simulink model "VCU10"  (R2021b)
settings: Solver=FixedStepDiscrete  StartTime=0.0  StopTime=10.0  FixedStep=0.01  RelTol=1e-3
values from neighbouring files (symbols this model uses):
  F = 0.0    [VCU10DB.sldd]
  FSEC_ESP_EMERGENCY_PRESSURE_MPA = 8.0    [VCU10DB.sldd]
  T = 1.0    [VCU10DB.sldd]
libraries: simulink x148, hdlsllib x90
(part 2 of 4)

== system VCU10/Motor_Control ==
  note: AS torque enable = ASMS AND AS_Driving AND R2D complete AND no Emergency lock.
  sensor_signal : Inport
  manual_driving_flag : Inport  Port=2
  as_flag : Inport  Port=3
  ipc_motor_torque : Inport  Port=4
  ts : Inport  Port=5
  function : TriggerPort  TriggerType=function-call  VariantControl=(inherit)
  ASTorque_Calculation : Subsystem
  AS_Driving_Read : DataStoreRead  DataStoreName=as_driving_flag  IndexOptions=Index vector (dialog)  Indices=1  OutputSizes=1
  AS_Emergency_Read : DataStoreRead  DataStoreName=as_emergency_flag  IndexOptions=Index vector (dialog)  Indices=1  OutputSizes=1
  AS_Torque_Enable : Logic  Inputs=4  AllPortsSameDT=off  OutDataTypeStr=boolean
  Emergency_Torque_Gate : Switch  Threshold=0.5
  Emergency_Zero_Torque : Constant  Value=0  OutDataTypeStr=double
  FSEC_Safety_Lock_Read : DataStoreRead  DataStoreName=safety_lock  IndexOptions=Index vector (dialog)  Indices=1  OutputSizes=1
  MCU1_Rx_Command : Subsystem
  MCU1_Rx_Command3 : Subsystem
  ManualTorque_Calculation : Subsystem
  Motor_Torque_Stateflow : Stateflow chart  TreatAsAtomicUnit=on
      settings: PortSchema="{\"entries\":[{\"content\":{\"sides\":[{\"content\":{\"connectorIds\":[\"In1\",\"In3\",\"In2\",\"In4\"]},\"type\":\"ConnectorPlacement.EquallySpacedRectSide\",\"uuid\":\"d9a8263c-4b6f-42da-8ac2-d6351ac22d7e\"},{\"content\":{\"connectorIds\":[\"Out1\"],\"side\":\"RIGHT\"},\"type\":\"ConnectorPlacement.EquallySpacedRectSide\",\"uuid\":\"5afddd84-d4d9-4932-bab9-0cf7e7557aa2\"},{\"content\":{\"connectorIds\":[],\"side\":\"TOP\"},\"type\":\"ConnectorPlacement.EquallySpacedRectSide\",\"uuid\":\"31244ac9-97b6-45b3-a8be-c5389c850836\"}]},\"type\":\"ConnectorPlacement.EquallySpacedConnector\",\"uuid\":\"4a9ac252-b735-4ae7-9487-f10bc9e5bec6\"}],\"packageUris\":[\"http://schema.mathworks.com/mf0/Connector/R2020b\"],\"version\":\"1.0\"}"
  No_FSEC_Safety_Lock : Logic  Operator=NOT  Inputs=1  AllPortsSameDT=off  OutDataTypeStr=boolean
  R2D_Complete : Logic  Operator=NOT  Inputs=1  AllPortsSameDT=off  OutDataTypeStr=boolean
  R2D_Read : DataStoreRead  DataStoreName=r2d_flag  IndexOptions=Index vector (dialog)  Indices=1  OutputSizes=1
  cana_motor_cmd : Outport
  cana_motor_cmd3 : Outport  Port=2
  wires:
  sensor_signal/1 -> ManualTorque_Calculation/1(sensor_signal)
  manual_driving_flag/1 -> Motor_Torque_Stateflow/1(manual_driving_flag)
  ManualTorque_Calculation/1(manual_torque) -> Motor_Torque_Stateflow/3(manual_torque)
  ASTorque_Calculation/1(as_torque) -> Motor_Torque_Stateflow/4(as_torque)
  ts/1 -> MCU1_Rx_Command/1(ts)
  [motor_torque] -> MCU1_Rx_Command/2(motor_torque)
  MCU1_Rx_Command/1(cana_motor_cmd) -> cana_motor_cmd/1
  MCU1_Rx_Command3/1(cana_motor_cmd3) -> cana_motor_cmd3/1
  ipc_motor_torque/1 -> ASTorque_Calculation/1(ipc_motor_torque)
  Emergency_Zero_Torque/1 -> Emergency_Torque_Gate/1
  AS_Emergency_Read/1 -> Emergency_Torque_Gate/2
  Motor_Torque_Stateflow/1(motor_torque) -> Emergency_Torque_Gate/3
  Emergency_Torque_Gate/1 -> [motor_torque]
  R2D_Read/1 -> R2D_Complete/1
  FSEC_Safety_Lock_Read/1 -> No_FSEC_Safety_Lock/1
  as_flag/1 -> AS_Torque_Enable/1
  AS_Driving_Read/1 -> AS_Torque_Enable/2
  R2D_Complete/1 -> AS_Torque_Enable/3
  No_FSEC_Safety_Lock/1 -> AS_Torque_Enable/4
  AS_Torque_Enable/1 -> Motor_Torque_Stateflow/2(as_task)

== system VCU10/Output_Convert ==
  note: Hardware mapping (netlist 2026-07-30): OUT1..7 = Brake, ASSI-B, ASSI-Y, EBS error, RES error, reserved, reserved; HO1..8 = EBS trigger, BMS, IMD, DI8, RUN, R2D, Emergency, reserved.
  led_brake : Inport
  led_assi_y : Inport  Port=2
  led_assi_b : Inport  Port=3
  led_ebserror : Inport  Port=4
  res_error : Inport  Port=5
  ebs_trig : Inport  Port=6
  led_bmserr : Inport  Port=7
  led_imderr : Inport  Port=8
  di8 : Inport  Port=9
  run : Inport  Port=10
  buzzer_r2d : Inport  Port=11
  buzzer_ebs : Inport  Port=12
  function : TriggerPort  TriggerType=function-call  VariantControl=(inherit)
  Physical_HO1_8_Pack : hdlsllib/Logic and Bit Operations/Bit Concat  numInputs=8
  Physical_OUT1_7_Pack : hdlsllib/Logic and Bit Operations/Bit Concat  numInputs=7
  Unused_HO_Bit : Constant  Value=false  OutDataTypeStr=boolean
  Unused_OUT_Bit : Constant  Value=false  OutDataTypeStr=boolean
  model_lox : Outport
  model_hox : Outport  Port=2
  wires:
  Unused_OUT_Bit/1 -> Physical_OUT1_7_Pack/1, Physical_OUT1_7_Pack/2
  res_error/1 -> Physical_OUT1_7_Pack/3
  led_ebserror/1 -> Physical_OUT1_7_Pack/4
  led_assi_y/1 -> Physical_OUT1_7_Pack/5
  led_assi_b/1 -> Physical_OUT1_7_Pack/6
  led_brake/1 -> Physical_OUT1_7_Pack/7
  Physical_OUT1_7_Pack/1 -> model_lox/1  "model_lox"
  Unused_HO_Bit/1 -> Physical_HO1_8_Pack/1
  buzzer_ebs/1 -> Physical_HO1_8_Pack/2
  buzzer_r2d/1 -> Physical_HO1_8_Pack/3
  run/1 -> Physical_HO1_8_Pack/4
  di8/1 -> Physical_HO1_8_Pack/5
  led_imderr/1 -> Physical_HO1_8_Pack/6
  led_bmserr/1 -> Physical_HO1_8_Pack/7
  ebs_trig/1 -> Physical_HO1_8_Pack/8
  Physical_HO1_8_Pack/1 -> model_hox/1  "model_hox"

== system VCU10/Res ==
  res_msg : Inport
  function : TriggerPort  TriggerType=function-call  VariantControl=(inherit)
  Bus Selector : BusSelector  OutputSignals=res_stop
  Res_Msg : Subsystem
  res_signal : Outport
  res_error : Outport  Port=2
  wires:
  res_msg/1 -> Res_Msg/1(res_msg)
  Res_Msg/1(res_signal) -> Bus Selector/1, res_signal/1
  Bus Selector/1 -> res_error/1  "<res_stop>"

== system VCU10/Sensor_Signal ==
  note: EBS气缸侧气压
  note: EBS气瓶侧气压
  note: FSEC diagnostics: brkps_raw is checked against 0.10-4.90 V. Air pressure sensor 1 is the reservoir/ready side; sensor 2 is the solenoid downstream/cylinder side.
  apps1 : Inport
  apps2 : Inport  Port=2
  brkps : Inport  Port=3
  airprs_sensor1 : Inport  Port=4
  airprs_sensor2 : Inport  Port=5
  wlspd_fsensor : Inport  Port=6
  wlspd_hsensor : Inport  Port=7
  function : TriggerPort  TriggerType=function-call  VariantControl=(inherit)
  1-D Lookup Table : Lookup_n-D  NumberOfTableDimensions=1  BreakpointsForDimension1=[252 2000]  IndexSearchMethod=Linear search  Table=[0.0 1.0]  ExtrapMethod=Clip  UseLastTableValue=on  InternalRulePriority=Speed  OutDataTypeStr=double  RndMeth=Simplest  InputSameDT=on
  1-D Lookup Table1 : Lookup_n-D  NumberOfTableDimensions=1  BreakpointsForDimension1=[252 2000]  IndexSearchMethod=Linear search  Table=[0.0 1.0]  ExtrapMethod=Clip  UseLastTableValue=on  InternalRulePriority=Speed  OutDataTypeStr=double  RndMeth=Simplest  InputSameDT=on
  1-D Lookup Table9 : Lookup_n-D  NumberOfTableDimensions=1  BreakpointsForDimension1=[252 2000]  IndexSearchMethod=Linear search  Table=[0.0 1.0]  ExtrapMethod=Clip  UseLastTableValue=on  InternalRulePriority=Speed  OutDataTypeStr=double  RndMeth=Simplest  InputSameDT=on
  Bus Creator : BusCreator  Inputs=12
  Data Type Conversion{,1..9,12,15} (12 alike) : DataTypeConversion  OutDataTypeStr=double
  Gain : Gain  Gain=single(0.001)
  Gain1 : Gain  Gain=single(0.001)
  Saturation : Saturate  UpperLimit=1  LowerLimit=0
  Saturation1 : Saturate  UpperLimit=1  LowerLimit=0
  Saturation2 : Saturate  UpperLimit=1  LowerLimit=0
  Subsystem : Subsystem
  sensor_signal : Outport
  wires:
  apps1/1 -> Data Type Conversion1/1, 1-D Lookup Table/1
  1-D Lookup Table/1 -> Data Type Conversion/1
  Data Type Conversion/1 -> Saturation/1
  Saturation/1 -> Bus Creator/1  "apps1_01"
  Data Type Conversion1/1 -> Bus Creator/2  "apps1_raw"
  Data Type Conversion2/1 -> Saturation1/1
  apps2/1 -> 1-D Lookup Table9/1, Data Type Conversion3/1
  1-D Lookup Table9/1 -> Data Type Conversion2/1
  Saturation1/1 -> Bus Creator/3  "apps2_01"
  Data Type Conversion3/1 -> Bus Creator/4  "apps2_raw"
  brkps/1 -> 1-D Lookup Table1/1, Data Type Conversion5/1
  1-D Lookup Table1/1 -> Data Type Conversion4/1
  Data Type Conversion4/1 -> Saturation2/1
  Saturation2/1 -> Bus Creator/5  "brkps"
  Data Type Conversion5/1 -> Bus Creator/6  "brkps_raw"
  wlspd_fsensor/1 -> Data Type Conversion6/1
  Data Type Conversion6/1 -> Subsystem/1(f_frequency)
  wlspd_hsensor/1 -> Data Type Conversion7/1
  Data Type Conversion7/1 -> Subsystem/2(h_frequency)
  Subsystem/1(wheel_speed_f) -> Data Type Conversion8/1
  Subsystem/2(wheel_speed_h) -> Data Type Conversion9/1
  Data Type Conversion8/1 -> Bus Creator/7  "wlspd_fsensor"
  Data Type Conversion9/1 -> Bus Creator/8  "wlspd_hsensor"
  Bus Creator/1 -> sensor_signal/1
  Data Type Conversion12/1 -> Bus Creator/9  "airprs_sensor1"
  airprs_sensor2/1 -> Gain1/1, Bus Creator/12  "airprs2_raw"
  Data Type Conversion15/1 -> Bus Creator/10  "airprs_sensor2"
  airprs_sensor1/1 -> Gain/1, Bus Creator/11  "airprs1_raw"
  Gain/1 -> Data Type Conversion12/1
  Gain1/1 -> Data Type Conversion15/1

== system VCU10/TS_Activation ==
  note: Software Emergency lock forces TS=0 until VCU low-voltage power cycle.
  note: AS Emergency forces TS=0 in the same model step; the software lock keeps TS off until VCU low-voltage power cycle.
  di8_out : Inport
  run_button : Inport  Port=2
  tsms_button : Inport  Port=3
  di8_in : Inport  Port=4
  as_flag : Inport  Port=5
  brake_on : Inport  Port=6
  function : TriggerPort  TriggerType=function-call  VariantControl=(inherit)
  AS_Emergency_Read : DataStoreRead  DataStoreName=as_emergency_flag  IndexOptions=Index vector (dialog)  Indices=1  OutputSizes=1
  Chart : Stateflow chart  TreatAsAtomicUnit=on
  Chart1 : Stateflow chart  TreatAsAtomicUnit=on
  Chart2 : Stateflow chart  TreatAsAtomicUnit=on
  FSEC_Safety_Lock_Read : DataStoreRead  DataStoreName=safety_lock  IndexOptions=Index vector (dialog)  Indices=1  OutputSizes=1
  Logical Operator : Logic  Operator=NOT  AllPortsSameDT=off  OutDataTypeStr=boolean
  Logical Operator1 : Logic  Operator=NOT  AllPortsSameDT=off  OutDataTypeStr=boolean
  Logical Operator2 : Logic  Operator=NOT  AllPortsSameDT=off  OutDataTypeStr=boolean
  No_AS_Emergency : Logic  Operator=NOT  Inputs=1  AllPortsSameDT=off  OutDataTypeStr=boolean
  No_FSEC_Safety_Lock : Logic  Operator=NOT  Inputs=1  AllPortsSameDT=off  OutDataTypeStr=boolean
  Switch : Switch  Criteria=u2 > Threshold
  TS_Safety_Gate : Logic  Inputs=3  AllPortsSameDT=off  OutDataTypeStr=boolean
  ts : Outport
  di8 : Outport  Port=2
  run : Outport  Port=3
  ts_warning : Outport  Port=4  OutDataTypeStr=boolean
  wires:
  di8_out/1 -> Logical Operator/1
  run_button/1 -> Logical Operator1/1
  Logical Operator1/1 -> Chart1/1(run_button)
  Chart/1(di8) -> di8/1, Chart2/1(di8)  "di8"
  Chart1/1(run) -> run/1, Chart2/2(run)  "run"
  tsms_button/1 -> Chart2/3(tsms_button)
  brake_on/1 -> Chart2/4(brake_on)
  as_flag/1 -> Chart2/5(as_flag), Switch/2
  di8_in/1 -> Logical Operator2/1
  Logical Operator/1 -> Switch/1
  Logical Operator2/1 -> Switch/3
  Switch/1 -> Chart/1(di8_button)
  Chart2/2(ts_warning) -> ts_warning/1
  FSEC_Safety_Lock_Read/1 -> No_FSEC_Safety_Lock/1
  Chart2/1(ts) -> TS_Safety_Gate/1
  No_FSEC_Safety_Lock/1 -> TS_Safety_Gate/2
  AS_Emergency_Read/1 -> No_AS_Emergency/1
  No_AS_Emergency/1 -> TS_Safety_Gate/3
  TS_Safety_Gate/1 -> ts/1

== system VCU10/AMI_CAN/AMI_Receivemsg ==
  AMI_Tx : Inport
  Bit Shift : hdlsllib/Logic and Bit Operations/Bit Shift  mode=Shift Right Logical  N=4
  Bitwise AND : simulink/Logic and Bit Operations/Bitwise Operator  logicop=AND  UseBitMask=on  BitMask=bin2dec('11110000')  BitMaskRealWorld=Stored Integer
  Demux : Demux  Outputs=8
  Terminator{,1..6} (7 alike) : Terminator
  ami_astask : Outport
  wires:
  Demux/6 -> Terminator3/1
  Demux/2 -> Terminator6/1
  Demux/4 -> Terminator1/1
  AMI_Tx/1 -> Demux/1
  Demux/7 -> Terminator4/1
  Demux/5 -> Terminator2/1
  Demux/8 -> Terminator5/1
  Demux/3 -> Terminator/1
  Demux/1 -> Bitwise AND/1
  Bitwise AND/1 -> Bit Shift/1
  Bit Shift/1 -> ami_astask/1

== system VCU10/AMI_CAN/AMI_Transmitmsg ==
  as_flag_state : Inport
  task_finish : Inport  Port=2
  Add1 : Sum
  Bit Shift : hdlsllib/Logic and Bit Operations/Bit Shift  mode=Shift Left Logical  N=1
  Bitwise AND : simulink/Logic and Bit Operations/Bitwise Operator  logicop=AND  UseBitMask=on  BitMask=bin2dec('01111111')  BitMaskRealWorld=Stored Integer
  Bus Selector : BusSelector  OutputSignals=as_off_flag,manual_driving_flag,as_ready_flag,r2d_flag,as_driving_flag,as_finished_flag,as_emergency_flag
  Chart : Stateflow chart  TreatAsAtomicUnit=on
  Ground{,1..6} (7 alike) : Ground
  Mux : Mux  Inputs=8
  Signal Conversion : SignalConversion  OverrideOpt=off
  AMI_RX : Outport
  wires:
  as_flag_state/1 -> Bus Selector/1
  Bitwise AND/1 -> Bit Shift/1
  Bit Shift/1 -> Add1/1
  task_finish/1 -> Add1/2
  Add1/1 -> Mux/1
  Bus Selector/1 -> Chart/1(as_off_flag)  "<as_off_flag>"
  Bus Selector/2 -> Chart/2(munual_driving_flag)  "<manual_driving_flag>"
  Bus Selector/3 -> Chart/3(as_ready_flag)  "<as_ready_flag>"
  Bus Selector/4 -> Chart/4(r2d_flag)  "<r2d_flag>"
  Bus Selector/5 -> Chart/5(as_driving_flag)  "<as_driving_flag>"
  Bus Selector/6 -> Chart/6(as_finished_flag)  "<as_finished_flag>"
  Bus Selector/7 -> Chart/7(as_emergency_flag)  "<as_emergency_flag>"
  Chart/1(ami_process) -> Bitwise AND/1
  Ground/1 -> Mux/2
  Ground1/1 -> Mux/3
  Ground2/1 -> Mux/4
  Ground3/1 -> Mux/5
  Ground4/1 -> Mux/6
  Ground5/1 -> Mux/7
  Ground6/1 -> Mux/8
  Mux/1 -> Signal Conversion/1
  Signal Conversion/1 -> AMI_RX/1

== system VCU10/ASB_Selfcheck/Brake_Sensor_Check ==
  note: 下四路为有效制动阈值油压
  note: 上四路油压信号阈值为非制动状态油压
  note: 所有常数待定
  airprs_sensor1 : Inport
  oilprs_frsensor : Inport  Port=2
  oilprs_rrsensor : Inport  Port=3
  oilprs_flsensor : Inport  Port=4
  oilprs_rlsensor : Inport  Port=5
  Compare To Constant : simulink/Logic and Bit Operations/Compare To Constant  relop=>=  const=3.5  OutDataTypeStr=boolean
  Compare To Constant{1,3,5,7} (4 alike) : simulink/Logic and Bit Operations/Compare To Constant  relop=>=  const=0.848  OutDataTypeStr=boolean
  Compare To Constant{2,4,6,8} (4 alike) : simulink/Logic and Bit Operations/Compare To Constant  relop=>=  const=0.742  OutDataTypeStr=boolean
  Logical Operator : Logic  Inputs=5  AllPortsSameDT=off  OutDataTypeStr=boolean
  Logical Operator1 : Logic  Inputs=4  AllPortsSameDT=off  OutDataTypeStr=boolean
  brksensor_check : Outport
  brake_on : Outport  Port=2
  wires:
  airprs_sensor1/1 -> Compare To Constant/1
  oilprs_frsensor/1 -> Compare To Constant5/1, Compare To Constant1/1
  oilprs_rrsensor/1 -> Compare To Constant7/1, Compare To Constant3/1
  oilprs_flsensor/1 -> Compare To Constant6/1, Compare To Constant2/1
  oilprs_rlsensor/1 -> Compare To Constant8/1, Compare To Constant4/1
  Compare To Constant3/1 -> Logical Operator/3
  Compare To Constant/1 -> Logical Operator/1
  Compare To Constant1/1 -> Logical Operator/2
  Compare To Constant2/1 -> Logical Operator/4
  Compare To Constant4/1 -> Logical Operator/5
  Logical Operator/1 -> brksensor_check/1
  Logical Operator1/1 -> brake_on/1
  Compare To Constant5/1 -> Logical Operator1/1
  Compare To Constant7/1 -> Logical Operator1/2
  Compare To Constant6/1 -> Logical Operator1/3
  Compare To Constant8/1 -> Logical Operator1/4

== system VCU10/AS_Stateflow/Car_Spdzero_Check ==
  wlspd_fsensor : Inport
  wlspd_hsensor : Inport  Port=2
  Compare To Constant : simulink/Logic and Bit Operations/Compare To Constant  relop===  const=0  OutDataTypeStr=boolean
  Compare To Constant1 : simulink/Logic and Bit Operations/Compare To Constant  relop===  const=0  OutDataTypeStr=boolean
  Dead Zone : DeadZone  SaturateOnIntegerOverflow=on
  Dead Zone1 : DeadZone  SaturateOnIntegerOverflow=on
  Logical Operator : Logic  AllPortsSameDT=off  OutDataTypeStr=boolean
  car_spdzero : Outport
  wires:
  wlspd_fsensor/1 -> Dead Zone/1
  wlspd_hsensor/1 -> Dead Zone1/1
  Dead Zone/1 -> Compare To Constant/1
  Dead Zone1/1 -> Compare To Constant1/1
  Compare To Constant/1 -> Logical Operator/1
  Compare To Constant1/1 -> Logical Operator/2
  Logical Operator/1 -> car_spdzero/1

== system VCU10/EPS/EPS_ReceiveMsg ==
  canb_epssendmsg1 : Inport
  canb_epssendmsg2 : Inport  Port=2
  EPS_Send_Msg1 : Subsystem
  EPS_Send_Msg2 : Subsystem
  canb_epssendmsg1signal : Outport
  canb_epssendmsg2signal : Outport  Port=2
  wires:
  canb_epssendmsg1/1 -> EPS_Send_Msg1/1(canb_epssendmsg1)
  EPS_Send_Msg1/1(canb_epssendmsg1signal) -> canb_epssendmsg1signal/1
  canb_epssendmsg2/1 -> EPS_Send_Msg2/1(canb_epssendmsg2)
  EPS_Send_Msg2/1(canb_epssendmsg2signal) -> canb_epssendmsg2signal/1

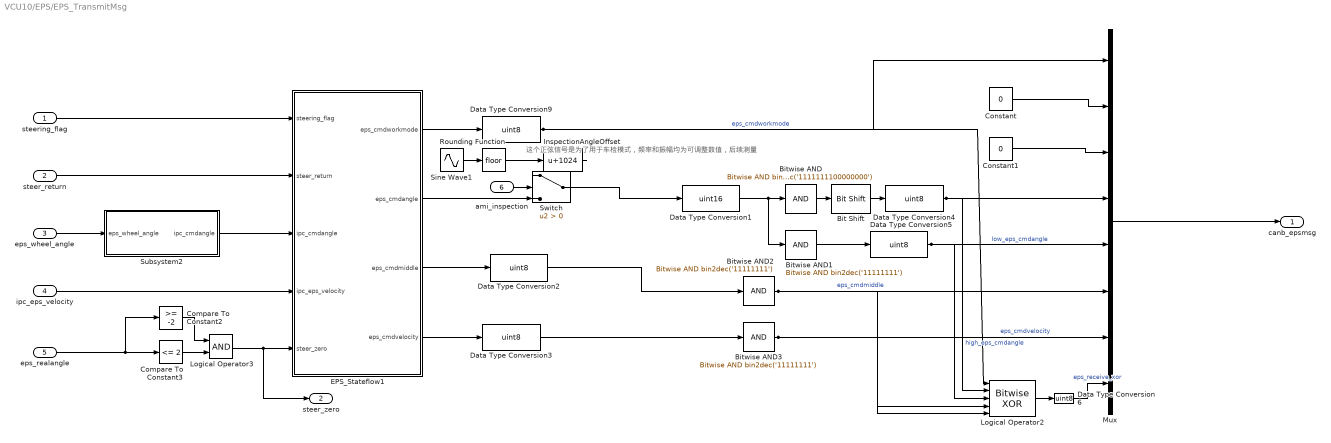
== system VCU10/EPS/EPS_TransmitMsg ==
  note: 这个正弦信号是为了用于车检模式，频率和振幅均为可调整数值，后续测量
  steering_flag : Inport
  steer_return : Inport  Port=2
  eps_wheel_angle : Inport  Port=3
  ipc_eps_velocity : Inport  Port=4
  eps_realangle : Inport  Port=5
  ami_inspection : Inport  Port=6
  Bit Shift : hdlsllib/Logic and Bit Operations/Bit Shift  mode=Shift Right Logical  N=8
  Bitwise AND : simulink/Logic and Bit Operations/Bitwise Operator  logicop=AND  UseBitMask=on  BitMask=bin2dec('1111111100000000')  BitMaskRealWorld=Stored Integer
  Bitwise AND1 : simulink/Logic and Bit Operations/Bitwise Operator  logicop=AND  UseBitMask=on  BitMask=bin2dec('11111111')  BitMaskRealWorld=Stored Integer
  Bitwise AND2 : simulink/Logic and Bit Operations/Bitwise Operator  logicop=AND  UseBitMask=on  BitMask=bin2dec('11111111')  BitMaskRealWorld=Stored Integer
  Bitwise AND3 : simulink/Logic and Bit Operations/Bitwise Operator  logicop=AND  UseBitMask=on  BitMask=bin2dec('11111111')  BitMaskRealWorld=Stored Integer
  Compare To Constant2 : simulink/Logic and Bit Operations/Compare To Constant  relop=>=  const=-2  OutDataTypeStr=boolean
  Compare To Constant3 : simulink/Logic and Bit Operations/Compare To Constant  relop=<=  const=2  OutDataTypeStr=boolean
  Constant : Constant  Value=0  OutDataTypeStr=uint8
  Constant1 : Constant  Value=0  OutDataTypeStr=uint8
  Data Type Conversion1 : DataTypeConversion  OutDataTypeStr=uint16
  Data Type Conversion{2..6,9} (6 alike) : DataTypeConversion  OutDataTypeStr=uint8
  EPS_Stateflow1 : Stateflow chart  TreatAsAtomicUnit=on
  InspectionAngleOffset : Bias  Bias=1024
  Logical Operator2 : simulink/Logic and Bit Operations/Bitwise Operator  logicop=XOR  UseBitMask=off  NumInputPorts=5  BitMask=bin2dec('11011001')  BitMaskRealWorld=Stored Integer
  Logical Operator3 : Logic  AllPortsSameDT=off  OutDataTypeStr=boolean
  Mux : Mux  Inputs=8
  Rounding Function : Rounding
  Sine Wave1 : Sin  Amplitude=90
  Subsystem2 : Subsystem
  Switch : Switch  Criteria=u2 > Threshold
  canb_epsmsg : Outport
  steer_zero : Outport  Port=2
  wires:
  Data Type Conversion5/1 -> Mux/5, Logical Operator2/3  "low_eps_cmdangle"
  Data Type Conversion9/1 -> Mux/1, Logical Operator2/1  "eps_cmdworkmode"
  Bitwise AND3/1 -> Mux/7, Logical Operator2/5  "eps_cmdvelocity"
  Compare To Constant3/1 -> Logical Operator3/2
  Data Type Conversion3/1 -> Bitwise AND3/1
  Bit Shift/1 -> Data Type Conversion4/1
  eps_realangle/1 -> Compare To Constant2/1, Compare To Constant3/1
  Data Type Conversion1/1 -> Bitwise AND/1, Bitwise AND1/1
  EPS_Stateflow1/4(eps_cmdvelocity) -> Data Type Conversion3/1
  Logical Operator3/1 -> steer_zero/1, EPS_Stateflow1/5(steer_zero)
  Bitwise AND2/1 -> Mux/6, Logical Operator2/4  "eps_cmdmiddle"
  EPS_Stateflow1/3(eps_cmdmiddle) -> Data Type Conversion2/1
  Constant1/1 -> Mux/3
  Bitwise AND/1 -> Bit Shift/1
  Data Type Conversion4/1 -> Mux/4, Logical Operator2/2  "high_eps_cmdangle"
  eps_wheel_angle/1 -> Subsystem2/1(eps_wheel_angle)
  Data Type Conversion2/1 -> Bitwise AND2/1
  Compare To Constant2/1 -> Logical Operator3/1
  steer_return/1 -> EPS_Stateflow1/2(steer_return)
  EPS_Stateflow1/1(eps_cmdworkmode) -> Data Type Conversion9/1
  Bitwise AND1/1 -> Data Type Conversion5/1
  ipc_eps_velocity/1 -> EPS_Stateflow1/4(ipc_eps_velocity)
  Constant/1 -> Mux/2
  Subsystem2/1(ipc_cmdangle) -> EPS_Stateflow1/3(ipc_cmdangle)
  Mux/1 -> canb_epsmsg/1
  steering_flag/1 -> EPS_Stateflow1/1(steering_flag)
  Switch/1 -> Data Type Conversion1/1
  Data Type Conversion6/1 -> Mux/8  "eps_receive_xor"
  ami_inspection/1 -> Switch/2
  EPS_Stateflow1/2(eps_cmdangle) -> Switch/3
  Sine Wave1/1 -> Rounding Function/1
  Logical Operator2/1 -> Data Type Conversion6/1
  Rounding Function/1 -> InspectionAngleOffset/1
  InspectionAngleOffset/1 -> Switch/1

== system VCU10/ESP/ESP_ReceiveMsg ==
  canb_esp_t01 : Inport
  canb_esp_t03 : Inport  Port=2
  canb_esp_t06 : Inport  Port=3
  canb_esp_t07 : Inport  Port=4
  Bus Selector : BusSelector  OutputSignals=lifeSig
  ESP_T_01 : Subsystem
  ESP_T_03 : Subsystem
  ESP_T_06 : Subsystem
  ESP_T_07 : Subsystem
  Subsystem : Subsystem
  ESP_T_01sigal : Outport
  ESP_T_03signal : Outport  Port=2
  ESP_T_06signal : Outport  Port=3
  ESP_T_07signal : Outport  Port=4
  brkmotor_check : Outport  Port=5
  wires:
  canb_esp_t01/1 -> ESP_T_01/1(canb_esp_t01)
  ESP_T_01/1(ESP_T_01sigal) -> ESP_T_01sigal/1
  canb_esp_t03/1 -> ESP_T_03/1(canb_esp_t03)
  canb_esp_t06/1 -> ESP_T_06/1(canb_esp_t06)
  ESP_T_06/1(ESP_T_06signal) -> ESP_T_06signal/1
  canb_esp_t07/1 -> ESP_T_07/1(canb_esp_t07)
  ESP_T_07/1(ESP_T_07signal) -> ESP_T_07signal/1
  Subsystem/1(brkmotor_check) -> brkmotor_check/1
  ESP_T_03/1(ESP_T_03signal) -> Bus Selector/1, ESP_T_03signal/1
  Bus Selector/1 -> Subsystem/1(lifesig)  "<lifeSig>"

== system VCU10/ESP/ESP_TransmitMsg ==
  ipc_esp_pressure : Inport
  brake_flag : Inport  Port=2
  lifeSig : Inport  Port=3
  checkSum : Inport  Port=4
  asms : Inport  Port=5  OutDataTypeStr=boolean
  ESP_R_00 : Subsystem
  canb_esp_r00 : Outport
  wires:
  ipc_esp_pressure/1 -> ESP_R_00/1(ipc_esp_pressure)
  brake_flag/1 -> ESP_R_00/2(brake_flag)
  ESP_R_00/1(canb_esp_r00) -> canb_esp_r00/1
  checkSum/1 -> ESP_R_00/4(checkSum)
  lifeSig/1 -> ESP_R_00/3(lifeSig)
  asms/1 -> ESP_R_00/5(asms)

== system VCU10/IPC/IPC_ReceiveMsg ==
  steer_return : Inport
  ipc_resgo : Inport  Port=2
  ipc_resstop : Inport  Port=3
  ipc_astask : Inport  Port=4
  IPC_Rx_Msg : Subsystem
  canb_ipcrxmsg : Outport
  wires:
  ipc_resgo/1 -> IPC_Rx_Msg/2(ipc_resgo)
  ipc_resstop/1 -> IPC_Rx_Msg/3(ipc_resstop)
  ipc_astask/1 -> IPC_Rx_Msg/4(ipc_astask)
  IPC_Rx_Msg/1(canb_ipcrxmsg) -> canb_ipcrxmsg/1
  steer_return/1 -> IPC_Rx_Msg/1(steer_return)

== system VCU10/IPC/IPC_TransmitMsg ==
  canb_ipctsmsg1 : Inport
  canb_ipctsmsg2 : Inport  Port=2
  IPC_Tx_Msg1 : Subsystem
  IPC_Tx_Msg2 : Subsystem
  ipc_esp_pressure : Outport
  ipc_motor_torque : Outport  Port=2
  ipc_eps_angle : Outport  Port=3
  ipc_eps_velocity : Outport  Port=4
  ipc_err : Outport  Port=5
  task_finish : Outport  Port=6
  ipc_heartbeat : Outport  Port=7
  ipc_lspd : Outport  Port=8
  ipc_hspd : Outport  Port=9
  wires:
  canb_ipctsmsg1/1 -> IPC_Tx_Msg1/1(canb_ipctsmsg1)
  IPC_Tx_Msg1/1(ipc_esp_pressure) -> ipc_esp_pressure/1
  IPC_Tx_Msg1/2(ipc_motor_torque) -> ipc_motor_torque/1
  canb_ipctsmsg2/1 -> IPC_Tx_Msg2/1(canb_ipctsmsg2)
  IPC_Tx_Msg2/2(ipc_eps_velocity) -> ipc_eps_velocity/1
  IPC_Tx_Msg2/1(ipc_eps_angle) -> ipc_eps_angle/1
  IPC_Tx_Msg2/3(ipc_err) -> ipc_err/1
  IPC_Tx_Msg2/4(task_finish) -> task_finish/1
  IPC_Tx_Msg2/6(ipc_lspd) -> ipc_lspd/1
  IPC_Tx_Msg2/5(ipc_heartbeat) -> ipc_heartbeat/1
  IPC_Tx_Msg2/7(ipc_hspd) -> ipc_hspd/1

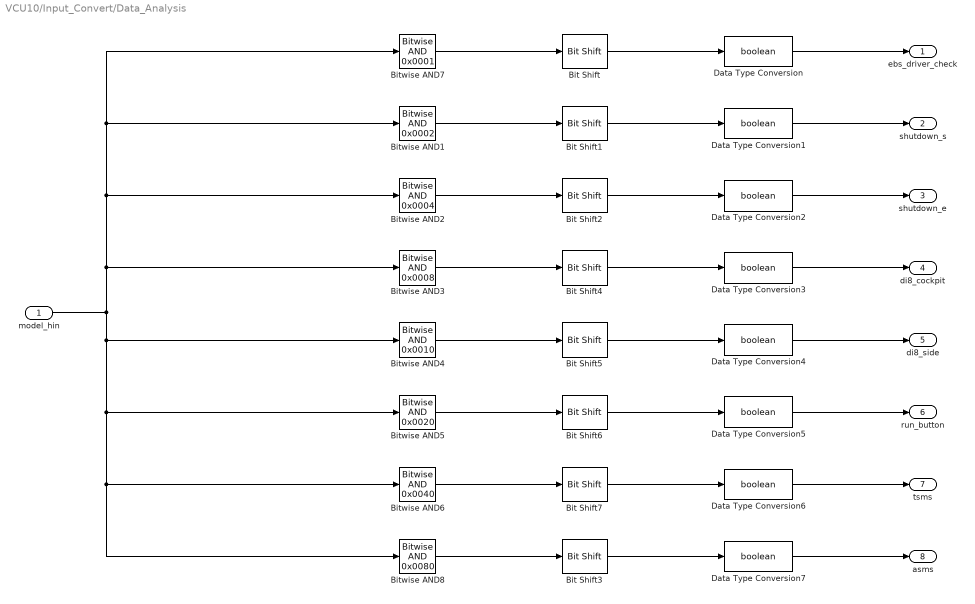
== system VCU10/Input_Convert/Data_Analysis ==
  model_hin : Inport
  Bit Shift : hdlsllib/Logic and Bit Operations/Bit Shift  mode=Shift Right Logical  N=0
  Bit Shift1 : hdlsllib/Logic and Bit Operations/Bit Shift  mode=Shift Right Logical  N=1
  Bit Shift2 : hdlsllib/Logic and Bit Operations/Bit Shift  mode=Shift Right Logical  N=2
  Bit Shift3 : hdlsllib/Logic and Bit Operations/Bit Shift  mode=Shift Right Logical  N=7
  Bit Shift4 : hdlsllib/Logic and Bit Operations/Bit Shift  mode=Shift Right Logical  N=3
  Bit Shift5 : hdlsllib/Logic and Bit Operations/Bit Shift  mode=Shift Right Logical  N=4
  Bit Shift6 : hdlsllib/Logic and Bit Operations/Bit Shift  mode=Shift Right Logical  N=5
  Bit Shift7 : hdlsllib/Logic and Bit Operations/Bit Shift  mode=Shift Right Logical  N=6
  Bitwise AND1 : simulink/Logic and Bit Operations/Bitwise Operator  logicop=AND  UseBitMask=on  BitMask=0x0002  BitMaskRealWorld=Stored Integer
  Bitwise AND2 : simulink/Logic and Bit Operations/Bitwise Operator  logicop=AND  UseBitMask=on  BitMask=0x0004  BitMaskRealWorld=Stored Integer
  Bitwise AND3 : simulink/Logic and Bit Operations/Bitwise Operator  logicop=AND  UseBitMask=on  BitMask=0x0008  BitMaskRealWorld=Stored Integer
  Bitwise AND4 : simulink/Logic and Bit Operations/Bitwise Operator  logicop=AND  UseBitMask=on  BitMask=0x0010  BitMaskRealWorld=Stored Integer
  Bitwise AND5 : simulink/Logic and Bit Operations/Bitwise Operator  logicop=AND  UseBitMask=on  BitMask=0x0020  BitMaskRealWorld=Stored Integer
  Bitwise AND6 : simulink/Logic and Bit Operations/Bitwise Operator  logicop=AND  UseBitMask=on  BitMask=0x0040  BitMaskRealWorld=Stored Integer
  Bitwise AND7 : simulink/Logic and Bit Operations/Bitwise Operator  logicop=AND  UseBitMask=on  BitMask=0x0001  BitMaskRealWorld=Stored Integer
  Bitwise AND8 : simulink/Logic and Bit Operations/Bitwise Operator  logicop=AND  UseBitMask=on  BitMask=0x0080  BitMaskRealWorld=Stored Integer
  Data Type Conversion{,1..7} (8 alike) : DataTypeConversion  OutDataTypeStr=boolean
  ebs_driver_check : Outport
  shutdown_s : Outport  Port=2
  shutdown_e : Outport  Port=3
  di8_cockpit : Outport  Port=4
  di8_side : Outport  Port=5
  run_button : Outport  Port=6
  tsms : Outport  Port=7
  asms : Outport  Port=8
  wires:
  Bitwise AND7/1 -> Bit Shift/1
  Bitwise AND1/1 -> Bit Shift1/1
  Bitwise AND2/1 -> Bit Shift2/1
  Bitwise AND3/1 -> Bit Shift4/1
  Bitwise AND4/1 -> Bit Shift5/1
  Bitwise AND5/1 -> Bit Shift6/1
  Bitwise AND6/1 -> Bit Shift7/1
  Bitwise AND8/1 -> Bit Shift3/1
  Bit Shift/1 -> Data Type Conversion/1
  Bit Shift1/1 -> Data Type Conversion1/1
  Bit Shift2/1 -> Data Type Conversion2/1
  Bit Shift4/1 -> Data Type Conversion3/1
  Bit Shift5/1 -> Data Type Conversion4/1
  Bit Shift6/1 -> Data Type Conversion5/1
  Bit Shift7/1 -> Data Type Conversion6/1
  Bit Shift3/1 -> Data Type Conversion7/1
  model_hin/1 -> Bitwise AND4/1, Bitwise AND6/1, Bitwise AND8/1, Bitwise AND5/1, Bitwise AND3/1, Bitwise AND2/1, Bitwise AND1/1, Bitwise AND7/1
  Data Type Conversion/1 -> ebs_driver_check/1
  Data Type Conversion3/1 -> di8_cockpit/1
  Data Type Conversion2/1 -> shutdown_e/1
  Data Type Conversion1/1 -> shutdown_s/1
  Data Type Conversion4/1 -> di8_side/1
  Data Type Conversion5/1 -> run_button/1
  Data Type Conversion6/1 -> tsms/1
  Data Type Conversion7/1 -> asms/1

== system VCU10/Input_Convert/Pedal_AinConvert_APP1 ==
  raw_data : Inport
  Data Type Conversion : DataTypeConversion  OutDataTypeStr=single
  Gain : Gain  Gain=single(187.5e-6)
  Saturation : Saturate  UpperLimit=5  LowerLimit=0
  real_vol : Outport
  wires:
  raw_data/1 -> Data Type Conversion/1
  Data Type Conversion/1 -> Gain/1
  Gain/1 -> Saturation/1
  Saturation/1 -> real_vol/1

== system VCU10/Input_Convert/Pedal_AinConvert_APP2 ==
  raw_data : Inport
  Data Type Conversion : DataTypeConversion  OutDataTypeStr=single
  Gain : Gain  Gain=single(187.5e-6)
  Saturation : Saturate  UpperLimit=5  LowerLimit=0
  real_vol : Outport
  wires:
  raw_data/1 -> Data Type Conversion/1
  Data Type Conversion/1 -> Gain/1
  Gain/1 -> Saturation/1
  Saturation/1 -> real_vol/1

== system VCU10/Input_Convert/Pedal_AinConvert_Brake ==
  raw_data : Inport
  Data Type Conversion : DataTypeConversion  OutDataTypeStr=single
  Gain : Gain  Gain=single(187.5e-6)
  Saturation : Saturate  UpperLimit=5  LowerLimit=0
  real_vol : Outport
  wires:
  raw_data/1 -> Data Type Conversion/1
  Data Type Conversion/1 -> Gain/1
  Gain/1 -> Saturation/1
  Saturation/1 -> real_vol/1

== system VCU10/Input_Convert/Pressure_AinConvert1 ==
  raw_data : Inport
  Data Type Conversion : DataTypeConversion  OutDataTypeStr=single
  Gain : Gain  Gain=single(0.0024169921875)
  Saturation : Saturate  UpperLimit=10  LowerLimit=0
  real_vol : Outport
  wires:
  raw_data/1 -> Data Type Conversion/1
  Data Type Conversion/1 -> Gain/1
  Gain/1 -> Saturation/1
  Saturation/1 -> real_vol/1

== system VCU10/Input_Convert/Pressure_AinConvert2 ==
  raw_data : Inport
  Data Type Conversion : DataTypeConversion  OutDataTypeStr=single
  Gain : Gain  Gain=single(0.0024169921875)
  Saturation : Saturate  UpperLimit=10  LowerLimit=0
  real_vol : Outport
  wires:
  raw_data/1 -> Data Type Conversion/1
  Data Type Conversion/1 -> Gain/1
  Gain/1 -> Saturation/1
  Saturation/1 -> real_vol/1

== system VCU10/LED_Control/EBS_LED ==
  note: 液压元件失效
  note: 手动阀未关
  note: 前气路故障
  note: 上电亮灯
  note: 气动元件检测与气压检测
  note: 油压检测
  note: 气缸侧气压在 EBS 未触发时可以接近 0 bar，不能单独作为断线故障。该传感器通过量程上限、两路合理性及触发后 200 ms 建压响应进行诊断。
  res_stop : Inport
  res_communication : Inport  Port=2
  Shutdown_Start : Inport  Port=3
  Shutdown_End : Inport  Port=4
  sensor_signal : Inport  Port=5
  ESP_T_03signal : Inport  Port=6
  asms_button : Inport  Port=7
  Bus Selector : BusSelector  OutputSignals=airprs_sensor1,airprs_sensor2
  Bus Selector1 : BusSelector  OutputSignals=oilprs_flsensor,oilprs_frsensor,oilprs_rlsensor,oilprs_rrsensor
  Compare To Constant : simulink/Logic and Bit Operations/Compare To Constant  relop=<=  const=1  OutDataTypeStr=boolean
  Compare To Constant2 : simulink/Logic and Bit Operations/Compare To Constant  relop=>=  const=3.5  OutDataTypeStr=boolean
  Compare To Constant{3..6} (4 alike) : simulink/Logic and Bit Operations/Compare To Constant  relop=<=  const=0.11  OutDataTypeStr=boolean
  Enabled Subsystem : Subsystem  TreatAsAtomicUnit=on
  Logical Operator : Logic  Operator=OR  Inputs=4  AllPortsSameDT=off  OutDataTypeStr=boolean
  Logical Operator2 : Logic  Inputs=4  AllPortsSameDT=off  OutDataTypeStr=boolean
  Logical Operator3 : Logic  Operator=OR  Inputs=4  AllPortsSameDT=off  OutDataTypeStr=boolean
  Shutdown_Button : Stateflow chart  TreatAsAtomicUnit=on
  display : Stateflow chart  TreatAsAtomicUnit=on
  led_ebs_error : Outport
  wires:
  Compare To Constant5/1 -> Logical Operator3/3
  Bus Selector/2 -> Compare To Constant2/1  "<airprs_sensor2>"
  Compare To Constant2/1 -> Enabled Subsystem/1(In1)
  Logical Operator/1 -> led_ebs_error/1
  Bus Selector1/4 -> Compare To Constant6/1  "<oilprs_rrsensor>"
  Compare To Constant4/1 -> Logical Operator3/2
  Bus Selector/1 -> Compare To Constant/1  "<airprs_sensor1>"
  Compare To Constant6/1 -> Logical Operator3/4
  Bus Selector1/1 -> Compare To Constant3/1  "<oilprs_flsensor>"
  asms_button/1 -> Logical Operator2/4
  Logical Operator2/1 -> Enabled Subsystem/Enable
  Shutdown_Button/1(shutdown_flag) -> Logical Operator2/3
  Compare To Constant3/1 -> Logical Operator3/1
  Bus Selector1/2 -> Compare To Constant4/1  "<oilprs_frsensor>"
  Bus Selector1/3 -> Compare To Constant5/1  "<oilprs_rlsensor>"
  ESP_T_03signal/1 -> Bus Selector1/1
  res_stop/1 -> Logical Operator2/1
  res_communication/1 -> Logical Operator2/2
  Shutdown_End/1 -> Shutdown_Button/2(Shutdown_End)
  Shutdown_Start/1 -> Shutdown_Button/1(Shutdown_Start)
  sensor_signal/1 -> Bus Selector/1
  Compare To Constant/1 -> Logical Operator/1
  Enabled Subsystem/1(Out1) -> Logical Operator/2
  Logical Operator3/1 -> Logical Operator/3
  display/1(spark) -> Logical Operator/4

== system VCU10/LED_Control/Subsystem ==
  as_led_blue : Inport
  asms_button : Inport  Port=2
  Constant : Constant  Value=0
  Constant1 : Constant  Value=0
  Constant2 : Constant
  Data Type Conversion : DataTypeConversion  OutDataTypeStr=boolean
  Pulse Generator : DiscretePulseGenerator  Period=50  PulseWidth=25  SampleTime=-1
  Switch : Switch  Criteria=u2 > Threshold  Threshold=10
  Switch1 : Switch  Criteria=u2 > Threshold  Threshold=10
  Switch2 : Switch  Criteria=u2 > Threshold  Threshold=40000
  blue : Stateflow chart  TreatAsAtomicUnit=on
  led_assi_blue : Outport
  wires:
  as_led_blue/1 -> blue/1(as_led_blue)
  Switch2/1 -> Data Type Conversion/1
  Switch/1 -> Switch2/2
  Constant2/1 -> Switch2/1
  [blue] -> Switch1/2
  Constant1/1 -> Switch1/3
  Data Type Conversion/1 -> led_assi_blue/1
  Switch1/1 -> Switch2/3
  [blue] -> Switch/1
  Pulse Generator/1 -> Switch1/1
  blue/1(blue) -> [blue]
  [blue] -> Switch/2
  Constant/1 -> Switch/3
  asms_button/1 -> blue/2(asms_button)

== system VCU10/LED_Control/Subsystem1 ==
  asms_button : Inport
  as_led_yellow : Inport  Port=2
  Constant : Constant  Value=0
  Constant1 : Constant  Value=0
  Constant3 : Constant
  Data Type Conversion : DataTypeConversion  OutDataTypeStr=boolean
  Pulse Generator : DiscretePulseGenerator  Period=50  PulseWidth=25  SampleTime=-1
  Switch : Switch  Criteria=u2 > Threshold  Threshold=10
  Switch1 : Switch  Criteria=u2 > Threshold  Threshold=10
  Switch2 : Switch  Criteria=u2 > Threshold  Threshold=40000
  yellow : Stateflow chart  TreatAsAtomicUnit=on
  led_assi_yellow : Outport
  wires:
  [yellow] -> Switch/2
  Switch1/1 -> Switch2/3
  Switch2/1 -> Data Type Conversion/1
  Constant3/1 -> Switch2/1
  yellow/1(yellow) -> [yellow]
  as_led_yellow/1 -> yellow/1(as_led_yellow)
  Switch/1 -> Switch2/2
  Pulse Generator/1 -> Switch1/1
  Data Type Conversion/1 -> led_assi_yellow/1
  [yellow] -> Switch1/2
  Constant/1 -> Switch/3
  [yellow] -> Switch/1
  Constant1/1 -> Switch1/3
  asms_button/1 -> yellow/2(asms_button)

== system VCU10/Motor_Control/ASTorque_Calculation ==
  ipc_motor_torque : Inport
  Data Type Conversion : DataTypeConversion  OutDataTypeStr=double
  Saturation : Saturate  UpperLimit=55  LowerLimit=0
  as_torque : Outport
  wires:
  ipc_motor_torque/1 -> Saturation/1
  Data Type Conversion/1 -> as_torque/1
  Saturation/1 -> Data Type Conversion/1

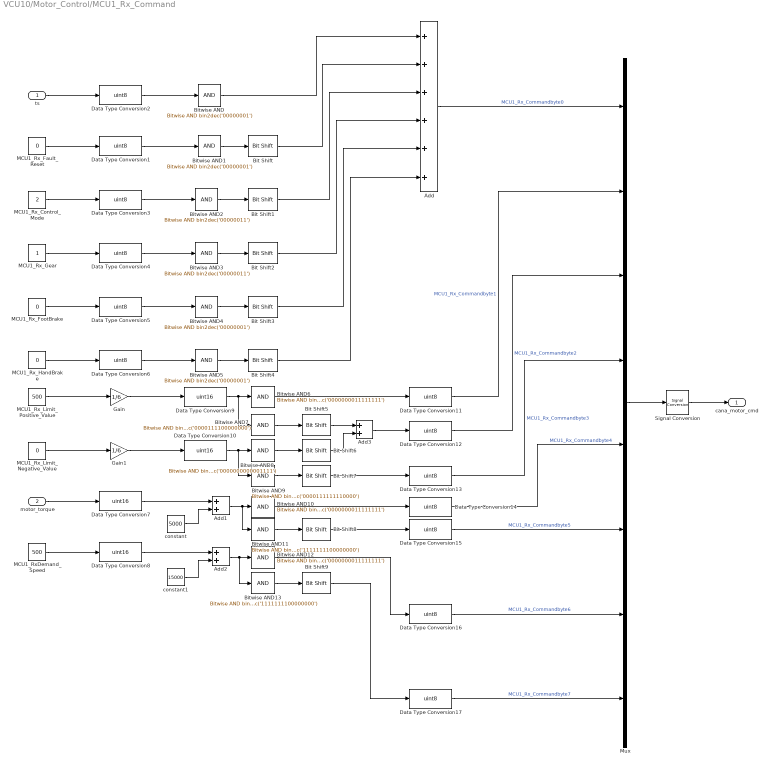
== system VCU10/Motor_Control/MCU1_Rx_Command ==
  ts : Inport
  motor_torque : Inport  Port=2
  Add : Sum  Inputs=++++++
  Add1 : Sum
  Add2 : Sum
  Add3 : Sum
  Bit Shift : hdlsllib/Logic and Bit Operations/Bit Shift  mode=Shift Left Logical  N=1
  Bit Shift1 : hdlsllib/Logic and Bit Operations/Bit Shift  mode=Shift Left Logical  N=2
  Bit Shift2 : hdlsllib/Logic and Bit Operations/Bit Shift  mode=Shift Left Logical  N=4
  Bit Shift3 : hdlsllib/Logic and Bit Operations/Bit Shift  mode=Shift Left Logical  N=6
  Bit Shift4 : hdlsllib/Logic and Bit Operations/Bit Shift  mode=Shift Left Logical  N=7
  Bit Shift5 : hdlsllib/Logic and Bit Operations/Bit Shift  mode=Shift Right Logical  N=8
  Bit Shift6 : hdlsllib/Logic and Bit Operations/Bit Shift  mode=Shift Left Logical  N=4
  Bit Shift7 : hdlsllib/Logic and Bit Operations/Bit Shift  mode=Shift Right Logical  N=4
  Bit Shift8 : hdlsllib/Logic and Bit Operations/Bit Shift  mode=Shift Right Logical  N=8
  Bit Shift9 : hdlsllib/Logic and Bit Operations/Bit Shift  mode=Shift Right Logical  N=8
  Bitwise AND{,1,4..5} (4 alike) : simulink/Logic and Bit Operations/Bitwise Operator  logicop=AND  UseBitMask=on  BitMask=bin2dec('00000001')  BitMaskRealWorld=Stored Integer
  Bitwise AND10 : simulink/Logic and Bit Operations/Bitwise Operator  logicop=AND  UseBitMask=on  BitMask=bin2dec('0000000011111111')  BitMaskRealWorld=Stored Integer
  Bitwise AND11 : simulink/Logic and Bit Operations/Bitwise Operator  logicop=AND  UseBitMask=on  BitMask=bin2dec('1111111100000000')  BitMaskRealWorld=Stored Integer
  Bitwise AND12 : simulink/Logic and Bit Operations/Bitwise Operator  logicop=AND  UseBitMask=on  BitMask=bin2dec('0000000011111111')  BitMaskRealWorld=Stored Integer
  Bitwise AND13 : simulink/Logic and Bit Operations/Bitwise Operator  logicop=AND  UseBitMask=on  BitMask=bin2dec('1111111100000000')  BitMaskRealWorld=Stored Integer
  Bitwise AND2 : simulink/Logic and Bit Operations/Bitwise Operator  logicop=AND  UseBitMask=on  BitMask=bin2dec('00000011')  BitMaskRealWorld=Stored Integer
  Bitwise AND3 : simulink/Logic and Bit Operations/Bitwise Operator  logicop=AND  UseBitMask=on  BitMask=bin2dec('00000011')  BitMaskRealWorld=Stored Integer
  Bitwise AND6 : simulink/Logic and Bit Operations/Bitwise Operator  logicop=AND  UseBitMask=on  BitMask=bin2dec('0000000011111111')  BitMaskRealWorld=Stored Integer
  Bitwise AND7 : simulink/Logic and Bit Operations/Bitwise Operator  logicop=AND  UseBitMask=on  BitMask=bin2dec('0000111100000000')  BitMaskRealWorld=Stored Integer
  Bitwise AND8 : simulink/Logic and Bit Operations/Bitwise Operator  logicop=AND  UseBitMask=on  BitMask=bin2dec('0000000000001111')  BitMaskRealWorld=Stored Integer
  Bitwise AND9 : simulink/Logic and Bit Operations/Bitwise Operator  logicop=AND  UseBitMask=on  BitMask=bin2dec('0000111111110000')  BitMaskRealWorld=Stored Integer
  Data Type Conversion{1..6,11..17} (13 alike) : DataTypeConversion  OutDataTypeStr=uint8
  Data Type Conversion{7..10} (4 alike) : DataTypeConversion  OutDataTypeStr=uint16
  Gain : Gain  Gain=1/6
  Gain1 : Gain  Gain=1/6
  MCU1_RxDemand_Speed : Constant  Value=500
  MCU1_Rx_Control_Mode : Constant  Value=2
  MCU1_Rx_Fault_Reset : Constant  Value=0
  MCU1_Rx_FootBrake : Constant  Value=0
  MCU1_Rx_Gear : Constant
  MCU1_Rx_HandBrake : Constant  Value=0
  MCU1_Rx_Limit_Negative_Value : Constant  Value=0  OutDataTypeStr=double
  MCU1_Rx_Limit_Positive_Value : Constant  Value=500  OutDataTypeStr=double
  Mux : Mux  Inputs=8
  Signal Conversion : SignalConversion  OverrideOpt=off
  constant : Constant  Value=5000  OutDataTypeStr=uint16
  constant1 : Constant  Value=15000  OutDataTypeStr=uint16
  cana_motor_cmd : Outport
  wires:
  ts/1 -> Data Type Conversion2/1
  MCU1_Rx_Fault_Reset/1 -> Data Type Conversion1/1
  MCU1_Rx_Control_Mode/1 -> Data Type Conversion3/1
  MCU1_Rx_Gear/1 -> Data Type Conversion4/1
  MCU1_Rx_FootBrake/1 -> Data Type Conversion5/1
  MCU1_Rx_HandBrake/1 -> Data Type Conversion6/1
  MCU1_Rx_Limit_Positive_Value/1 -> Gain/1
  MCU1_Rx_Limit_Negative_Value/1 -> Gain1/1
  MCU1_RxDemand_Speed/1 -> Data Type Conversion8/1
  Data Type Conversion2/1 -> Bitwise AND/1
  Data Type Conversion1/1 -> Bitwise AND1/1
  Bitwise AND1/1 -> Bit Shift/1
  Data Type Conversion3/1 -> Bitwise AND2/1
  Bitwise AND2/1 -> Bit Shift1/1
  Data Type Conversion4/1 -> Bitwise AND3/1
  Bitwise AND3/1 -> Bit Shift2/1
  Data Type Conversion5/1 -> Bitwise AND4/1
  Bitwise AND4/1 -> Bit Shift3/1
  Data Type Conversion6/1 -> Bitwise AND5/1
  Bitwise AND5/1 -> Bit Shift4/1
  Bitwise AND/1 -> Add/1
  Bit Shift/1 -> Add/2
  Bit Shift1/1 -> Add/3
  Bit Shift2/1 -> Add/4
  Bit Shift3/1 -> Add/5
  Bit Shift4/1 -> Add/6
  Add/1 -> Mux/1  "MCU1_Rx_Commandbyte0"
  motor_torque/1 -> Data Type Conversion7/1
  Data Type Conversion7/1 -> Add1/1
  constant/1 -> Add1/2
  Data Type Conversion8/1 -> Add2/1
  constant1/1 -> Add2/2
  Gain/1 -> Data Type Conversion9/1
  Data Type Conversion9/1 -> Bitwise AND7/1, Bitwise AND6/1
  Bitwise AND6/1 -> Data Type Conversion11/1
  Bitwise AND7/1 -> Bit Shift5/1
  Gain1/1 -> Data Type Conversion10/1
  Data Type Conversion10/1 -> Bitwise AND9/1, Bitwise AND8/1
  Data Type Conversion11/1 -> Mux/2  "MCU1_Rx_Commandbyte1"
  Bit Shift5/1 -> Add3/1
  Bitwise AND8/1 -> Bit Shift6/1
  Bit Shift6/1 -> Add3/2
  Add3/1 -> Data Type Conversion12/1
  Data Type Conversion12/1 -> Mux/3  "MCU1_Rx_Commandbyte2"
  Bitwise AND9/1 -> Bit Shift7/1
  Bit Shift7/1 -> Data Type Conversion13/1
  Data Type Conversion13/1 -> Mux/4  "MCU1_Rx_Commandbyte3"
  Add1/1 -> Bitwise AND11/1, Bitwise AND10/1
  Bitwise AND10/1 -> Data Type Conversion14/1
  Data Type Conversion14/1 -> Mux/5  "MCU1_Rx_Commandbyte4"
  Bitwise AND11/1 -> Bit Shift8/1
  Bit Shift8/1 -> Data Type Conversion15/1
  Data Type Conversion15/1 -> Mux/6  "MCU1_Rx_Commandbyte5"
  Bit Shift9/1 -> Data Type Conversion17/1
  Bitwise AND13/1 -> Bit Shift9/1
  Bitwise AND12/1 -> Data Type Conversion16/1
  Add2/1 -> Bitwise AND13/1, Bitwise AND12/1
  Data Type Conversion16/1 -> Mux/7  "MCU1_Rx_Commandbyte6"
  Data Type Conversion17/1 -> Mux/8  "MCU1_Rx_Commandbyte7"
  Mux/1 -> Signal Conversion/1
  Signal Conversion/1 -> cana_motor_cmd/1

== system VCU10/Motor_Control/MCU1_Rx_Command3 ==
  Bit Shift : hdlsllib/Logic and Bit Operations/Bit Shift  mode=Shift Right Logical  N=8
  Bit Shift1 : hdlsllib/Logic and Bit Operations/Bit Shift  mode=Shift Right Logical  N=8
  Bitwise AND : simulink/Logic and Bit Operations/Bitwise Operator  logicop=AND  UseBitMask=on  BitMask=bin2dec('0000000011111111')  BitMaskRealWorld=Stored Integer
  Bitwise AND1 : simulink/Logic and Bit Operations/Bitwise Operator  logicop=AND  UseBitMask=on  BitMask=bin2dec('1111111100000000')  BitMaskRealWorld=Stored Integer
  Bitwise AND2 : simulink/Logic and Bit Operations/Bitwise Operator  logicop=AND  UseBitMask=on  BitMask=bin2dec('0000000011111111')  BitMaskRealWorld=Stored Integer
  Bitwise AND3 : simulink/Logic and Bit Operations/Bitwise Operator  logicop=AND  UseBitMask=on  BitMask=bin2dec('1111111100000000')  BitMaskRealWorld=Stored Integer
  Data Type Conversion1 : DataTypeConversion  OutDataTypeStr=uint16
  Data Type Conversion{2..4,6} (4 alike) : DataTypeConversion  OutDataTypeStr=uint8
  Data Type Conversion5 : DataTypeConversion  OutDataTypeStr=uint16
  Mux : Mux  Inputs=8
  constant : Constant  Value=0  OutDataTypeStr=uint8
  f32__speed_KI : Constant  Value=9.3
  f32__speed_KP : Constant  Value=93
  cana_motor_cmd3 : Outport
  wires:
  f32__speed_KP/1 -> Data Type Conversion5/1
  f32__speed_KI/1 -> Data Type Conversion1/1
  Data Type Conversion5/1 -> Bitwise AND1/1, Bitwise AND/1
  Bitwise AND/1 -> Data Type Conversion2/1
  Data Type Conversion2/1 -> Mux/1  "MCU1_Rx_Command3byte0"
  Bit Shift/1 -> Data Type Conversion3/1
  Bitwise AND1/1 -> Bit Shift/1
  Data Type Conversion3/1 -> Mux/2  "MCU1_Rx_Command3byte1"
  Bitwise AND2/1 -> Data Type Conversion4/1
  Bit Shift1/1 -> Data Type Conversion6/1
  Data Type Conversion6/1 -> Mux/4  "MCU1_Rx_Command3byte3"
  Data Type Conversion1/1 -> Bitwise AND3/1, Bitwise AND2/1
  Data Type Conversion4/1 -> Mux/3  "MCU1_Rx_Command3byte2"
  Bitwise AND3/1 -> Bit Shift1/1
  constant/1 -> Mux/8, Mux/7, Mux/6, Mux/5
  Mux/1 -> cana_motor_cmd3/1

== system VCU10/Motor_Control/ManualTorque_Calculation ==
  note: APPS：双通道差值仍按 10% 检查；任一原始 ADC 低于 0.10 V 或高于 4.90 V 时立即将转矩置零，100 ms 确认故障，连续正常 500 ms 恢复。阈值需在踏板最终标定后复核。
  sensor_signal : Inport
  APPS_Electrical_Monitor : MATLAB Function  TreatAsAtomicUnit=on
  APPS_Fault_Terminator : Terminator
  APPS_Torque_Valid_Gate : Logic  AllPortsSameDT=off  OutDataTypeStr=boolean
  Add : Sum
  Bus Selector : BusSelector  OutputSignals=apps1_01,apps2_01,apps1_raw,apps2_raw
  Constant : Constant  Value=2
  Constant1 : Constant  Value=0
  Divide : Product  Inputs=*/
  Logical Operator : Logic  Operator=NOT  AllPortsSameDT=off  OutDataTypeStr=boolean
  Pedal_Fault_Check : Stateflow chart  TreatAsAtomicUnit=on
  Product : Product
  Switch : Switch  Criteria=u2 > Threshold
  max_torque : Constant  Value=50
  manual_torque : Outport
  wires:
  Constant1/1 -> Switch/3
  Switch/1 -> manual_torque/1
  max_torque/1 -> Product/2
  sensor_signal/1 -> Bus Selector/1
  Bus Selector/1 -> Add/1, Pedal_Fault_Check/1(apps1)  "<apps1_01>"
  Bus Selector/2 -> Pedal_Fault_Check/2(apps2), Add/2  "<apps2_01>"
  Divide/1 -> Product/1
  Product/1 -> Switch/1
  Constant/1 -> Divide/2
  Pedal_Fault_Check/1(pedal_error) -> Logical Operator/1
  Add/1 -> Divide/1
  Bus Selector/3 -> APPS_Electrical_Monitor/1(apps1_raw_mv)  "<apps1_raw>"
  Bus Selector/4 -> APPS_Electrical_Monitor/2(apps2_raw_mv)  "<apps2_raw>"
  Logical Operator/1 -> APPS_Torque_Valid_Gate/1
  APPS_Electrical_Monitor/1(apps_valid) -> APPS_Torque_Valid_Gate/2
  APPS_Torque_Valid_Gate/1 -> Switch/2
  APPS_Electrical_Monitor/2(apps_electrical_fault) -> APPS_Fault_Terminator/1

== system VCU10/Res/Res_Msg ==
  res_msg : Inport
  Bit Shift : hdlsllib/Logic and Bit Operations/Bit Shift  mode=Shift Right Logical  N=1
  Bit Shift1 : hdlsllib/Logic and Bit Operations/Bit Shift  mode=Shift Right Logical  N=2
  Bit Shift2 : hdlsllib/Logic and Bit Operations/Bit Shift  mode=Shift Right Logical  N=4
  Bitwise AND : simulink/Logic and Bit Operations/Bitwise Operator  logicop=AND  UseBitMask=on  BitMask=bin2dec('00000001')  BitMaskRealWorld=Stored Integer
  Bitwise AND1 : simulink/Logic and Bit Operations/Bitwise Operator  logicop=AND  UseBitMask=on  BitMask=bin2dec('00000010')  BitMaskRealWorld=Stored Integer
  Bitwise AND2 : simulink/Logic and Bit Operations/Bitwise Operator  logicop=AND  UseBitMask=on  BitMask=bin2dec('00000100')  BitMaskRealWorld=Stored Integer
  Bitwise AND3 : simulink/Logic and Bit Operations/Bitwise Operator  logicop=AND  UseBitMask=on  BitMask=bin2dec('00010000')  BitMaskRealWorld=Stored Integer
  Bitwise AND4 : simulink/Logic and Bit Operations/Bitwise Operator  logicop=AND  UseBitMask=on  BitMask=bin2dec('11111111')  BitMaskRealWorld=Stored Integer
  Bitwise AND5 : simulink/Logic and Bit Operations/Bitwise Operator  logicop=AND  UseBitMask=on  BitMask=bin2dec('11111111')  BitMaskRealWorld=Stored Integer
  Bus Creator : BusCreator  Inputs=5
  Data Type Conversion{1..3,7} (4 alike) : DataTypeConversion  OutDataTypeStr=boolean
  Demux : Demux  Outputs=8
  Logical Operator : simulink/Logic and Bit Operations/Bitwise Operator  logicop=XOR  UseBitMask=off  NumInputPorts=2  BitMask=bin2dec('11011001')  BitMaskRealWorld=Stored Integer
  Stop_Checksum_Match : RelationalOperator  Operator===  OutDataTypeStr=boolean  RndMeth=Simplest
  Subsystem : Subsystem
  Terminator{,1..4} (5 alike) : Terminator
  Validated_Stop : Logic  Inputs=3  AllPortsSameDT=off  OutDataTypeStr=boolean
  res_signal : Outport
  wires:
  res_msg/1 -> Demux/1
  Demux/1 -> Bitwise AND/1, Bitwise AND1/1, Bitwise AND2/1, Bitwise AND3/1, Logical Operator/1
  Bitwise AND/1 -> Data Type Conversion7/1
  Bitwise AND1/1 -> Bit Shift/1
  Bit Shift/1 -> Data Type Conversion1/1
  Bitwise AND2/1 -> Bit Shift1/1
  Data Type Conversion1/1 -> Bus Creator/2  "res_gobutton"
  Bit Shift1/1 -> Data Type Conversion2/1
  Data Type Conversion2/1 -> Subsystem/1(res_communication), Bus Creator/3  "res_communication"
  Bitwise AND3/1 -> Bit Shift2/1
  Bit Shift2/1 -> Data Type Conversion3/1
  Data Type Conversion3/1 -> Bus Creator/4  "res_go"
  Demux/2 -> Bitwise AND4/1, Logical Operator/2
  Bitwise AND4/1 -> Subsystem/2(res_heartbeat)  "res_heartbeat"
  Demux/3 -> Bitwise AND5/1
  Bitwise AND5/1 -> Subsystem/3(res_xorcheck), Stop_Checksum_Match/1  "res_xorcheck"
  Demux/5 -> Terminator/1
  Demux/4 -> Terminator1/1
  Demux/6 -> Terminator2/1
  Demux/7 -> Terminator3/1
  Demux/8 -> Terminator4/1
  Bus Creator/1 -> res_signal/1
  Subsystem/1(res_check) -> Bus Creator/5, Validated_Stop/2  "res_check"
  Logical Operator/1 -> Subsystem/4(xor_consequence), Stop_Checksum_Match/2  "xor_consequence"
  Data Type Conversion7/1 -> Validated_Stop/1  "res_stop"
  Stop_Checksum_Match/1 -> Validated_Stop/3
  Validated_Stop/1 -> Bus Creator/1  "res_stop"

== system VCU10/Sensor_Signal/Subsystem ==
  note: % u为频率，r为车轮滚动半径y=u*36.0*pi/180.0*0.225*3.6
  f_frequency : Inport
  h_frequency : Inport  Port=2
  Constant : Constant  Value=180
  Constant1 : Constant  Value=0.225
  Constant2 : Constant  Value=3.6
  Constant3 : Constant  Value=180
  Divide : Product  Inputs=*/
  Divide1 : Product  Inputs=*/
  Gain : Gain  Gain=36
  Gain1 : Gain  Gain=3.1415
  Gain2 : Gain  Gain=36
  Gain3 : Gain  Gain=3.1415
  Product : Product
  Product1 : Product
  Product2 : Product
  wheel_speed_f : Outport
  wheel_speed_h : Outport  Port=2
  wires:
  f_frequency/1 -> Gain/1
  Gain/1 -> Gain1/1
  Gain1/1 -> Divide/1
  Constant1/1 -> Product/1
  Constant2/1 -> Product/2
  Constant/1 -> Divide/2
  Divide/1 -> Product1/1
  Product/1 -> Product2/1, Product1/2
  Product1/1 -> wheel_speed_f/1
  h_frequency/1 -> Gain2/1
  Gain2/1 -> Gain3/1
  Constant3/1 -> Divide1/2
  Gain3/1 -> Divide1/1
  Product2/1 -> wheel_speed_h/1
  Divide1/1 -> Product2/2

== system VCU10/EPS/EPS_ReceiveMsg/EPS_Send_Msg1 ==
  canb_epssendmsg1 : Inport
  Add : Sum  Inputs=-++
  Add1 : Sum  Inputs=+-
  Bus Creator : BusCreator  Inputs=7
  Constant : Constant  Value=12.8  OutDataTypeStr=double
  Constant1 : Constant  Value=1024  OutDataTypeStr=double
  Data Type Conversion{1..3,9} (4 alike) : DataTypeConversion  OutDataTypeStr=double
  Demux : Demux  Outputs=8
  Gain1 : Gain  Gain=256
  TorqueScale : Gain  Gain=0.1
  canb_epssendmsg1signal : Outport
  wires:
  canb_epssendmsg1/1 -> Demux/1
  Bus Creator/1 -> canb_epssendmsg1signal/1
  Demux/1 -> Bus Creator/1  "eps_workmode"
  Demux/2 -> Data Type Conversion9/1
  Demux/3 -> Bus Creator/3  "eps_errorcode1"
  Data Type Conversion3/1 -> Bus Creator/4  "eps_realangle"
  Demux/7 -> Bus Creator/6  "eps_errorcode2"
  Demux/8 -> Bus Creator/7  "eps_sned_xor"
  Data Type Conversion9/1 -> TorqueScale/1
  Constant/1 -> Add1/2
  Add1/1 -> Bus Creator/2  "eps_torque"
  Data Type Conversion1/1 -> Gain1/1
  Constant1/1 -> Add/1
  Data Type Conversion2/1 -> Add/3
  Add/1 -> Data Type Conversion3/1
  Gain1/1 -> Add/2  "eps_realangle"
  TorqueScale/1 -> Add1/1
  Demux/4 -> Data Type Conversion1/1  "eps_midddlefeedback"
  Demux/5 -> Data Type Conversion2/1
  Demux/6 -> Bus Creator/5  "eps_midddlefeedback"
